simulink model "PROJ_Cga"  (R2020a)
settings: Solver=FixedStepAuto  StartTime=0.0  StopTime=2  FixedStep=1e-6  RelTol=1e-3  EnableMultiTasking=on
libraries: powerlib x18
settings Model: SimulationMode=accelerator  Creator=SINA  LastModifiedBy=ABO-CHIFA
settings DataIOCC: ReturnWorkspaceOutputs=off
settings OptimizationCC: LifeSpan=inf
settings DebuggingCC: AlgebraicLoopMsg=none  ArtificialAlgebraicLoopMsg=none  MaxConsecutiveZCsMsg=none  ModelReferenceExtraNoncontSigs=none  OperatingPointInterfaceChecksumMismatchMsg=none  SFUnexpectedBacktrackingDiag=warning  SFNoUnconditionalDefaultTransitionDiag=warning  ArithmeticOperatorsInVariantConditions=warning
settings SFSimCC: SimUseLocalCustomCode=off  CustomCodeUndefinedFunction=UseInterfaceOnly
settings RTWCC: RTWUseLocalCustomCode=off
settings CodeAppCC: StateflowObjectComments=on
settings GRTTargetCC: TargetLangStandard=C89/C90 (ANSI)
settings ConfigComp: CovMetricSettings=dw  CovHtmlReporting=on  CovSaveCumulativeToWorkspaceVar=on  CovSaveSingleToWorkspaceVar=on  CovExternalEMLEnable=off
settings SimscapeCC: SimscapeNormalizeSystem=off

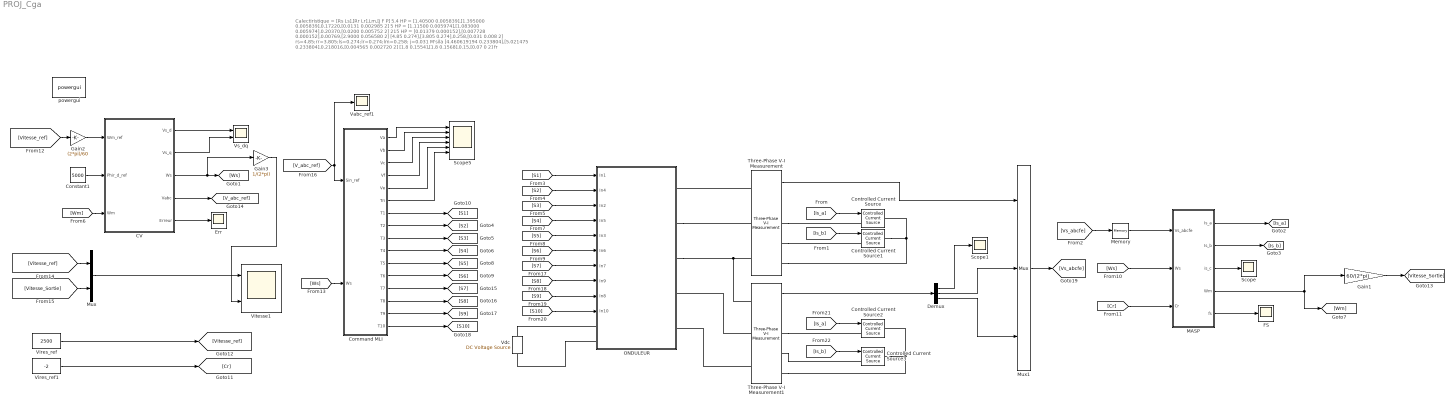
== system PROJ_Cga ==
  note: Calectiristique = [Rs Ls],[Rr Lr],Lm,[J F P]
      |
      | 5.4 HP = [1.40500 0.005839],[1.395000 0.005839],0.17220,[0.0131 0.002985 2]
      | 5 HP = [1.11500 0.005974],[1.083000 0.005974],0.20370,[0.0200 0.005752 2]
      | 215 HP = [0.01379 0.000152],[0.007728 0.000152],0.00769,[2.9000 0.056580 2]
      | [4.85 0.274],[3.805 0.274],0.258,[0.031 0.008 2]
      | rs=4.85;rr=3.805;ls=0.274;lr=0.274;lm=0.258;
      | j=0.031
      |
      | M'sila
      | [4.460619194 0.233804],[5.021475 0.233804],0.218016,[0.004565 0.002720 2]
      |
      | [1.8 0.1554],[1.8 0.1568],0.15,[0.07 0 2] fr
  CV : Subsystem
  Command MLI : Subsystem
  Constant1 : Constant  Value=5000
  Controlled Current Source{,1..3} (4 alike) : powerlib/Electrical Sources/Controlled Current Source  Initialize=off  Source_Type=AC  Amplitude=0  Phase=0  Frequency=50  Measurements=None
  Demux : Demux  Outputs=3
  Err : Scope
  FS : Scope
  Gain1 : Gain  Gain=60/(2*pi)
  Gain2 : Gain  Gain=(2*pi)/60
  Gain3 : Gain  Gain=1/(2*pi)
  MASP : Subsystem
  Memory : Memory
  Mux : Mux  Inputs=2
  Mux1 : Mux  Inputs=3
  ONDULEUR : Subsystem
  Scope : Scope
  Scope1 : Scope
  Scope5 : Scope  NumInputPorts=6
  Three-Phase V-I Measurement : powerlib/Measurements/Three-Phase V-I Measurement  VoltageMeasurement=phase-to-phase  SetLabelV=off  LabelV=Vabc  Vpu=off  VpuLL=off  CurrentMeasurement=yes  SetLabelI=off  LabelI=Iabc  Ipu=off  Pbase=100e6  Vbase=500e3  OutputType=Complex  PhasorSimulation=off  PSBequivalent=0
  Three-Phase V-I Measurement1 : powerlib/Measurements/Three-Phase V-I Measurement  VoltageMeasurement=phase-to-phase  SetLabelV=off  LabelV=Vabc  Vpu=off  VpuLL=off  CurrentMeasurement=yes  SetLabelI=off  LabelI=Iabc  Ipu=off  Pbase=100e6  Vbase=500e3  OutputType=Complex  PhasorSimulation=off  PSBequivalent=0
  "Vabc_ref1 " : Scope
  Vdc : powerlib/Electrical Sources/DC Voltage Source  Amplitude=650  Measurements=Voltage
  Vires_ref : Constant  Value=2500
  Vires_ref1 : Constant  Value=-2
  Vitesse1 : Scope  NumInputPorts=2
  Vs_dq : Scope  NumInputPorts=2
  powergui : powerlib/powergui  Priority=1  SimulationMode=Discrete  SampleTime=1e-6  frequency=60  Iterations=50  frequencyindice=0  Pbase=100e6  ErrMax=1e-4  UnitsV=kV  UnitsW=MW  buscounter=0  FunctionMessages=off  echomessages=off  EnableUseOfTLC=off  CurrentSourceSwitches=off  DisableSnubberDevices=off  DisableRonSwitches=off  DisableVfSwitches=off  DisplayEquations=off  AutomaticDiscreteSolvers=off  SolverType=Tustin/Backward Euler (TBE)  Interpol=off  ExternalGateDelay=off  methode=off  Ts=0  x0status=blocks  SPID=off  SwTol=0  HookPort=off  NonlinearTolerance=1e-4  nMaxIteration=100  ContinueOnMaxIteration=off  RestoreLinks=warning  ResistiveCurrentMeasurement=off  Frange=[0:2:500]  Ylog=off  Xlog=on  ShowGrid=off  save=off  variable=ZData  structure=0  ZoomFFT=on  StartTime=0.0  cycles=1  DisplayStyle=1  fundamental=60  FreqAxis=off  MaxFrequency=1000  frequencyindicesteady=1  RmsSteady=1  display=off
  wires:
  [Vs_abcfe] -> Memory/1
  Command MLI/12(T6) -> [S6]
  Command MLI/11(T5) -> [S5]
  Command MLI/10(T4) -> [S4]
  Command MLI/9(T3) -> [S3]
  Command MLI/8(T2) -> [S2]
  Command MLI/7(T1) -> [S1]
  Memory/1 -> MASP/1(Vs_abcfe)
  MASP/1(Is_a) -> [Is_a]
  MASP/2(Is_b) -> [Is_b]
  Constant1/1 -> CV/2(Phir_d_ref)
  Gain2/1 -> CV/1(Wm_ref)
  [Ws] -> MASP/2(Ws)
  Vires_ref1/1 -> [Cr]
  [Cr] -> MASP/3(Cr)
  [Ws] -> Command MLI/2(Ws)
  [Vitesse_ref] -> Gain2/1
  MASP/4(Wm) -> Gain1/1, [Wm]
  Gain1/1 -> [Vitesse_Sortie]
  CV/5(Erreur) -> Err/1
  CV/1(Vs_d) -> Vs_dq/1
  CV/2(Vs_q) -> Vs_dq/2
  [Wm] -> CV/3(Wm)
  MASP/5(fs) -> FS/1
  [Vitesse_Sortie] -> Mux/2
  [Vitesse_ref] -> Mux/1
  Mux/1 -> Vitesse1/1
  Vires_ref/1 -> [Vitesse_ref]
  CV/4(Vabc) -> [V_abc_ref]
  [V_abc_ref] -> "Vabc_ref1 "/1, Command MLI/1(Sin_ref)
  CV/3(Ws) -> Gain3/1, [Ws]
  Command MLI/1(Va) -> Scope5/1
  Command MLI/2(Vb) -> Scope5/2
  Command MLI/3(Vc) -> Scope5/3
  Command MLI/4(Vf) -> Scope5/4
  Command MLI/5(Ve) -> Scope5/5
  Command MLI/6(Tri) -> Scope5/6
  Command MLI/13(T7) -> [S7]
  Command MLI/14(T8) -> [S8]
  Command MLI/15(T9) -> [S9]
  Command MLI/16(T10) -> [S10]
  [S1] -> ONDULEUR/1(In1)
  [S2] -> ONDULEUR/2(In4)
  [S3] -> ONDULEUR/3(In2)
  [S4] -> ONDULEUR/4(In5)
  [S5] -> ONDULEUR/5(In3)
  [S6] -> ONDULEUR/6(In6)
  [S7] -> ONDULEUR/7(In7)
  [S8] -> ONDULEUR/8(In9)
  [S9] -> ONDULEUR/9(In8)
  [S10] -> ONDULEUR/10(In10)
  Mux1/1 -> [Vs_abcfe]
  MASP/3(is_c) -> Scope/1
  Demux/2 -> Mux1/2
  Demux/3 -> Mux1/3
  [Is_a] -> Controlled Current Source/1
  [Is_b] -> Controlled Current Source1/1
  [Is_a] -> Controlled Current Source2/1
  [Is_b] -> Controlled Current Source3/1
  Three-Phase V-I Measurement1/1 -> Demux/1
  Three-Phase V-I Measurement/1 -> Mux1/1
  Demux/1 -> Scope1/1
  Gain3/1 -> Vitesse1/2
  connections:
  Vdc/RConn1 -- ONDULEUR/LConn1
  ONDULEUR/LConn2 -- Vdc/LConn1
  Three-Phase V-I Measurement/LConn1 -- ONDULEUR/RConn1
  ONDULEUR/RConn2 -- Three-Phase V-I Measurement/LConn2
  ONDULEUR/RConn3 -- Three-Phase V-I Measurement1/LConn1 -- Three-Phase V-I Measurement/LConn3
  Three-Phase V-I Measurement1/LConn2 -- ONDULEUR/RConn4
  Three-Phase V-I Measurement1/LConn3 -- ONDULEUR/RConn5
  Three-Phase V-I Measurement/RConn1 -- Controlled Current Source/LConn1
  Three-Phase V-I Measurement/RConn2 -- Controlled Current Source1/LConn1
  Three-Phase V-I Measurement/RConn3 -- Controlled Current Source1/RConn1 -- Controlled Current Source/RConn1
  Three-Phase V-I Measurement1/RConn1 -- Controlled Current Source2/LConn1
  Three-Phase V-I Measurement1/RConn2 -- Controlled Current Source3/LConn1
  Three-Phase V-I Measurement1/RConn3 -- Controlled Current Source3/RConn1 -- Controlled Current Source2/RConn1

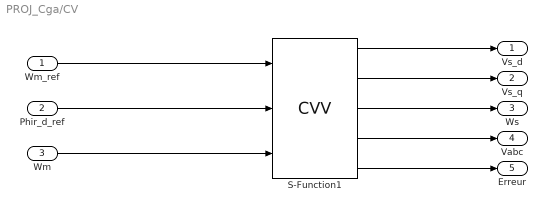
== system PROJ_Cga/CV ==
  Wm_ref : Inport
  Phir_d_ref : Inport  Port=2
  Wm : Inport  Port=3
  S-Function1 : S-Function  FunctionName=CVV  Parameters=[1.40500 0.005839],[1.395000 0.005839],0.17220,[0.0131 0.002985 2]  SFunctionDeploymentMode=off  EnableBusSupport=off
  Vs_d : Outport
  Vs_q : Outport  Port=2
  Ws : Outport  Port=3
  Vabc : Outport  Port=4
  Erreur : Outport  Port=5
  wires:
  S-Function1/4 -> Vabc/1
  S-Function1/3 -> Ws/1
  S-Function1/2 -> Vs_q/1
  S-Function1/1 -> Vs_d/1
  Wm/1 -> S-Function1/3
  Phir_d_ref/1 -> S-Function1/2
  Wm_ref/1 -> S-Function1/1
  S-Function1/5 -> Erreur/1

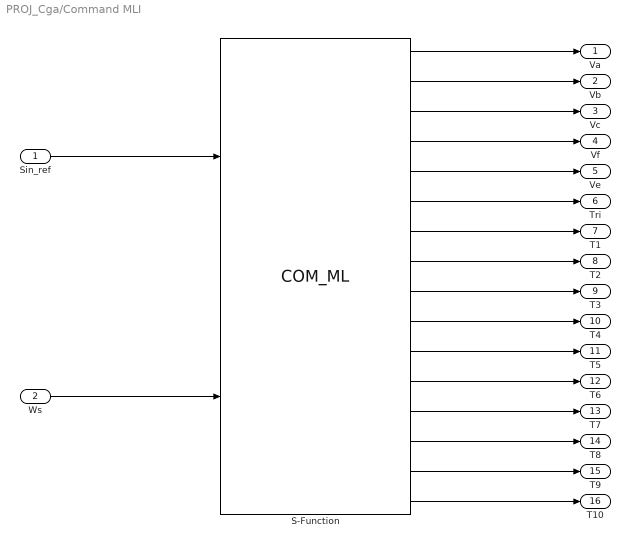
== system PROJ_Cga/Command MLI ==
  Sin_ref : Inport
  Ws : Inport  Port=2
  S-Function : S-Function  FunctionName=COM_ML  SFunctionDeploymentMode=off  EnableBusSupport=off
  Va : Outport
  Vb : Outport  Port=2
  Vc : Outport  Port=3
  Vf : Outport  Port=4
  Ve : Outport  Port=5
  Tri : Outport  Port=6
  T1 : Outport  Port=7
  T2 : Outport  Port=8
  T3 : Outport  Port=9
  T4 : Outport  Port=10
  T5 : Outport  Port=11
  T6 : Outport  Port=12
  T7 : Outport  Port=13
  T8 : Outport  Port=14
  T9 : Outport  Port=15
  T10 : Outport  Port=16
  wires:
  Sin_ref/1 -> S-Function/1
  Ws/1 -> S-Function/2
  S-Function/1 -> Va/1
  S-Function/2 -> Vb/1
  S-Function/3 -> Vc/1
  S-Function/4 -> Vf/1
  S-Function/5 -> Ve/1
  S-Function/6 -> Tri/1
  S-Function/7 -> T1/1
  S-Function/8 -> T2/1
  S-Function/9 -> T3/1
  S-Function/10 -> T4/1
  S-Function/11 -> T5/1
  S-Function/12 -> T6/1
  S-Function/13 -> T7/1
  S-Function/14 -> T8/1
  S-Function/15 -> T9/1
  S-Function/16 -> T10/1

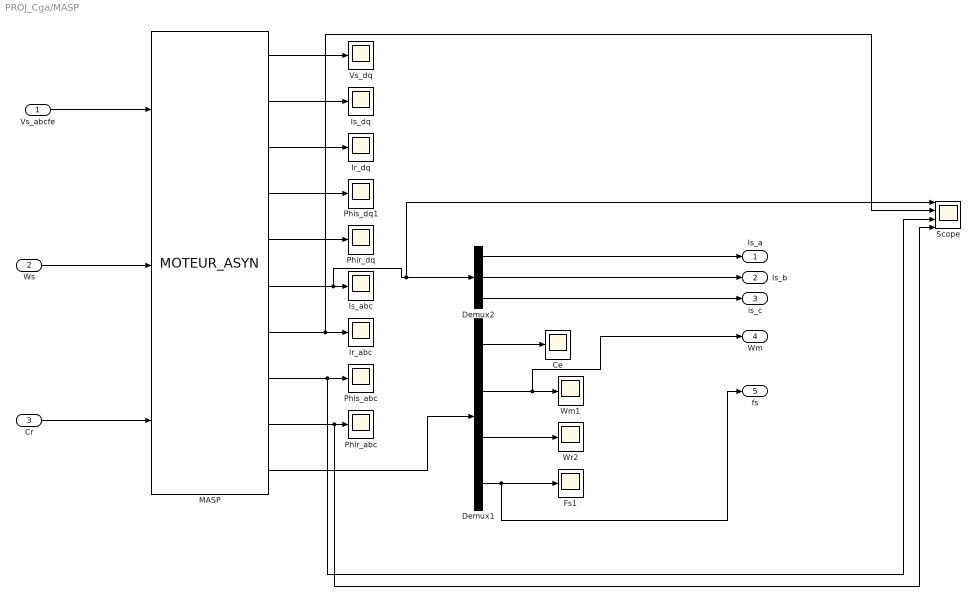
== system PROJ_Cga/MASP ==
  Vs_abcfe : Inport
  Ws : Inport  Port=2
  Cr : Inport  Port=3
  Ce : Scope
  Demux1 : Demux
  Demux2 : Demux  Outputs=3
  Fs1 : Scope
  Ir_abc : Scope
  Ir_dq : Scope
  Is_abc : Scope
  Is_dq : Scope
  MASP : S-Function  FunctionName=MOTEUR_ASYN  Parameters=[1.40500 0.005839],[1.395000 0.005839],0.17220,[0.0131 0.002985 2]  SFunctionDeploymentMode=off  EnableBusSupport=off
  Phir_abc : Scope
  Phir_dq : Scope
  Phis_abc : Scope
  Phis_dq1 : Scope
  Scope : Scope  NumInputPorts=4
  Vs_dq : Scope
  Wm1 : Scope
  Wr2 : Scope
  Is_a : Outport
  Is_b : Outport  Port=2
  is_c : Outport  Port=3
  Wm : Outport  Port=4
  fs : Outport  Port=5
  wires:
  Cr/1 -> MASP/3
  Demux1/1 -> Ce/1
  Vs_abcfe/1 -> MASP/1
  Demux2/2 -> Is_b/1
  MASP/4 -> Phis_dq1/1
  MASP/1 -> Vs_dq/1
  MASP/8 -> Scope/3, Phis_abc/1
  MASP/5 -> Phir_dq/1
  MASP/10 -> Demux1/1
  MASP/3 -> Ir_dq/1
  MASP/6 -> Scope/1, Demux2/1, Is_abc/1
  Demux1/4 -> fs/1, Fs1/1
  MASP/2 -> Is_dq/1
  MASP/9 -> Scope/4, Phir_abc/1
  MASP/7 -> Scope/2, Ir_abc/1
  Demux2/3 -> is_c/1
  Demux2/1 -> Is_a/1
  Ws/1 -> MASP/2
  Demux1/3 -> Wr2/1
  Demux1/2 -> Wm/1, Wm1/1

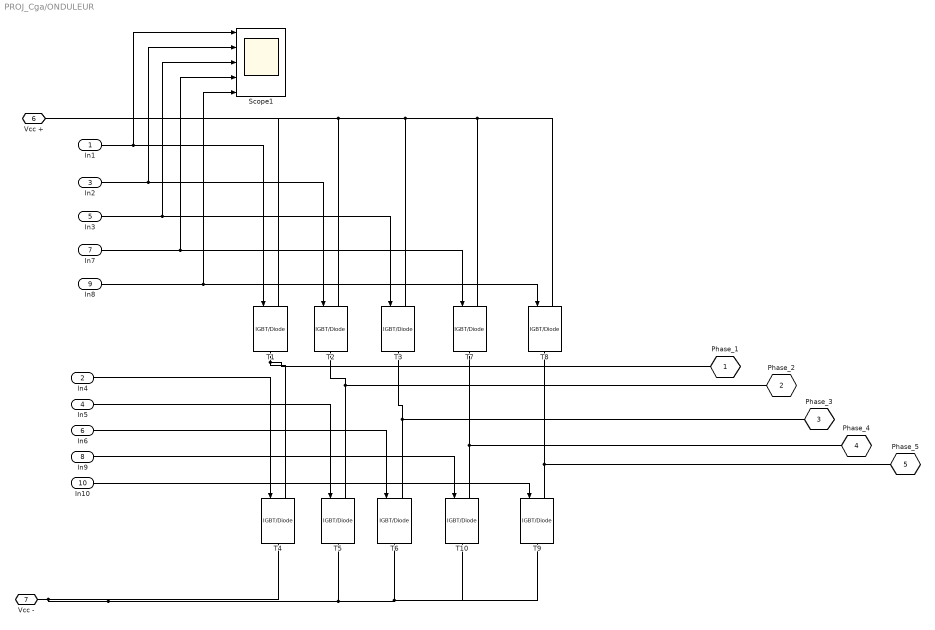
== system PROJ_Cga/ONDULEUR ==
  In1 : Inport
  In4 : Inport  Port=2
  In2 : Inport  Port=3
  In5 : Inport  Port=4
  In3 : Inport  Port=5
  In6 : Inport  Port=6
  In7 : Inport  Port=7
  In9 : Inport  Port=8
  In8 : Inport  Port=9
  In10 : Inport  Port=10
  Scope1 : Scope  NumInputPorts=5
  T{1..10} (10 alike) : powerlib/Power Electronics/IGBT//Diode  Ron=1e-3  Rs=1e5  Cs=inf  Measurements=off
  Phase_1 : PMIOPort  Tag=PMCPort  Side=Right
  Phase_2 : PMIOPort  Tag=PMCPort  Port=2  Side=Right
  Phase_3 : PMIOPort  Tag=PMCPort  Port=3  Side=Right
  Phase_4 : PMIOPort  Tag=PMCPort  Port=4  Side=Right
  Phase_5 : PMIOPort  Tag=PMCPort  Port=5  Side=Right
  Vcc + : PMIOPort  Port=6  Side=Left
  Vcc - : PMIOPort  Port=7  Side=Left
  wires:
  In1/1 -> Scope1/1, T1/1
  In9/1 -> T10/1
  In5/1 -> T5/1
  In4/1 -> T4/1
  In3/1 -> Scope1/3, T3/1
  In8/1 -> Scope1/5, T8/1
  In7/1 -> Scope1/4, T7/1
  In10/1 -> T9/1
  In6/1 -> T6/1
  In2/1 -> Scope1/2, T2/1
  connections:
  T6/LConn1 -- T3/RConn1 -- Phase_3/RConn1
  T5/LConn1 -- T2/RConn1 -- Phase_2/RConn1
  Phase_4/RConn1 -- T10/LConn1 -- T7/RConn1
  Vcc -/RConn1 -- T10/RConn1 -- T9/RConn1 -- T6/RConn1 -- T5/RConn1 -- T4/RConn1
  T7/LConn1 -- T8/LConn1 -- T3/LConn1 -- Vcc +/RConn1 -- T1/LConn1 -- T2/LConn1
  T9/LConn1 -- Phase_5/RConn1 -- T8/RConn1
  T1/RConn1 -- T4/LConn1 -- Phase_1/RConn1
